simulink model "cdip_odq_sim"  (R2013a)
settings: Solver=ode4  SolverMode=SingleTasking  StartTime=0.0  StopTime=t_end  FixedStep=0.001  RelTol=1e-3
values from neighbouring files (symbols this model uses):
  dtheta_0 = 0    [p2c234_ex1_cdip_odq.m]    (also in p2c234_ex1_cdip_odq_custom.m; p2c244_ex3_cdip_sampled_data_lqr_sim.m; p2c244_ex3_cdip_sampled_data_lqr_sim_custom.m)
  dz_0 = 0    [p2c234_ex1_cdip_odq.m]    (also in p2c234_ex1_cdip_odq_custom.m; p2c244_ex3_cdip_sampled_data_lqr_sim.m; p2c244_ex3_cdip_sampled_data_lqr_sim_custom.m)
  K = - lqr(A,B,Q,R)    [p2c234_ex1_cdip_odq.m]    (also in p2c234_ex1_cdip_odq_custom.m; p2c244_ex3_cdip_sampled_data_lqr_sim.m; p2c244_ex3_cdip_sampled_data_lqr_sim_custom.m)
  theta_0 = pi/18    (= 0.174532925199)    [p2c234_ex1_cdip_odq.m]    (also in p2c234_ex1_cdip_odq_custom.m; p2c244_ex3_cdip_sampled_data_lqr_sim.m = 0.261799387799; p2c244_ex3_cdip_sampled_data_lqr_sim_custom.m = 0.261799387799)
  ts = 0.01    [p2c234_ex1_cdip_odq.m]    (also in p2c234_ex1_cdip_odq_custom.m; p2c242_ex2_cart_ipd.m = 0.025; p2c242_ex2_cart_ipd_custom.m = 0.025; p2c244_ex3_cdip_sampled_data_lqr_sim.m = 0.1)
  z_0 = 0    [p2c234_ex1_cdip_odq.m]    (also in p2c234_ex1_cdip_odq_custom.m; p2c244_ex3_cdip_sampled_data_lqr_sim.m; p2c244_ex3_cdip_sampled_data_lqr_sim_custom.m)
undefined symbols (not defined in the file or in its folder): ac, bc, g, Jp, lp, mp, mup, Sigma_Q
libraries: odqblock x1
settings Model: Creator=kawata  LastModifiedBy=kawata
settings SolverCC: AutoInsertRateTranBlk=on  InsertRTBMode=Always
settings DataIOCC: LimitDataPoints=off  SignalLoggingSaveFormat=ModelDataLogs
settings OptimizationCC: ExpressionDepthLimit=2147483647
settings DebuggingCC: FcnCallInpInsideContextMsg=UseLocalSettings
settings GRTTargetCC: CombineOutputUpdateFcns=off  GRTInterface=on

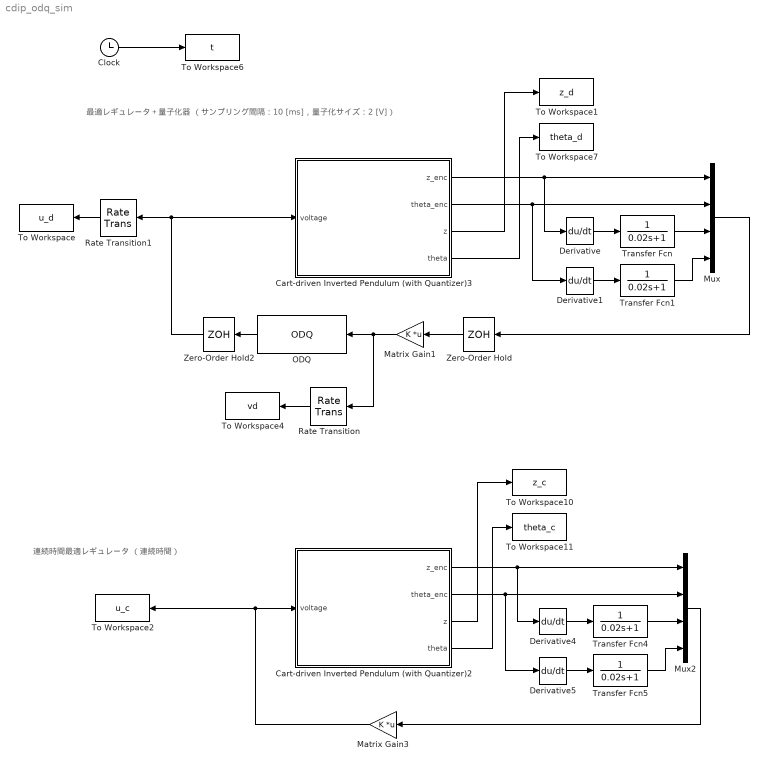
== system cdip_odq_sim ==
  note: 最適レギュレータ＋量子化器
      | （サンプリング間隔：10 [ms]，量子化サイズ：2 [V]）
  note: 連続時間最適レギュレータ
      | （連続時間）
  Cart-driven Inverted Pendulum (with Quantizer)2 : Subsystem
      mask Display: image(imread('cdip_photo.jpg'),'center')
  Cart-driven Inverted Pendulum (with Quantizer)3 : Subsystem
      mask Display: image(imread('cdip_photo.jpg'),'center')
  Clock : Clock
  Derivative{,1,4..5} (4 alike) : Derivative
  Matrix Gain1 : Gain  Gain=K  Multiplication=Matrix(K*u)  SaturateOnIntegerOverflow=on  OutDataTypeStr=Inherit: Same as input  ParamDataTypeStr=Inherit: Same as input
  Matrix Gain3 : Gain  Gain=K  Multiplication=Matrix(K*u)  SaturateOnIntegerOverflow=on  OutDataTypeStr=Inherit: Same as input  ParamDataTypeStr=Inherit: Same as input
  Mux : Mux
  Mux2 : Mux
  ODQ : odqblock/ODQ  A=Sigma_Q.a  B1=Sigma_Q.b1  B2=Sigma_Q.b2  C=Sigma_Q.c  d=d  Ts=ts
  Rate Transition : RateTransition  OutPortSampleTime=0.001
  Rate Transition1 : RateTransition  OutPortSampleTime=0.001
  To Workspace : ToWorkspace  VariableName=u_d  SampleTime=-1
  To Workspace1 : ToWorkspace  VariableName=z_d  SampleTime=-1
  To Workspace10 : ToWorkspace  VariableName=z_c  SampleTime=-1
  To Workspace11 : ToWorkspace  VariableName=theta_c  SampleTime=-1
  To Workspace2 : ToWorkspace  VariableName=u_c  SampleTime=0.001
  To Workspace4 : ToWorkspace  VariableName=vd  SampleTime=-1
  To Workspace6 : ToWorkspace  VariableName=t  SampleTime=-1
  To Workspace7 : ToWorkspace  VariableName=theta_d  SampleTime=-1
  Transfer Fcn{,1,4..5} (4 alike) : TransferFcn  Denominator=[0.02 1]
  Zero-Order Hold : ZeroOrderHold  SampleTime=ts
  Zero-Order Hold2 : ZeroOrderHold  SampleTime=ts
  wires:
  Zero-Order Hold/1 -> Matrix Gain1/1
  Zero-Order Hold2/1 -> Cart-driven Inverted Pendulum (with Quantizer)3/1(voltage), Rate Transition1/1
  Clock/1 -> To Workspace6/1
  ODQ/1 -> Zero-Order Hold2/1
  Matrix Gain1/1 -> ODQ/1, Rate Transition/1
  Rate Transition1/1 -> To Workspace/1
  Rate Transition/1 -> To Workspace4/1
  Mux/1 -> Zero-Order Hold/1
  Cart-driven Inverted Pendulum (with Quantizer)3/1(z_enc) -> Derivative/1, Mux/1
  Cart-driven Inverted Pendulum (with Quantizer)3/2(theta_enc) -> Derivative1/1, Mux/2
  Derivative/1 -> Transfer Fcn/1
  Transfer Fcn/1 -> Mux/3
  Transfer Fcn1/1 -> Mux/4
  Cart-driven Inverted Pendulum (with Quantizer)3/3(z) -> To Workspace1/1
  Cart-driven Inverted Pendulum (with Quantizer)3/4(theta) -> To Workspace7/1
  Derivative1/1 -> Transfer Fcn1/1
  Mux2/1 -> Matrix Gain3/1
  Matrix Gain3/1 -> To Workspace2/1, Cart-driven Inverted Pendulum (with Quantizer)2/1(voltage)
  Cart-driven Inverted Pendulum (with Quantizer)2/1(z_enc) -> Derivative4/1, Mux2/1
  Cart-driven Inverted Pendulum (with Quantizer)2/2(theta_enc) -> Derivative5/1, Mux2/2
  Derivative4/1 -> Transfer Fcn4/1
  Derivative5/1 -> Transfer Fcn5/1
  Transfer Fcn4/1 -> Mux2/3
  Transfer Fcn5/1 -> Mux2/4
  Cart-driven Inverted Pendulum (with Quantizer)2/3(z) -> To Workspace10/1
  Cart-driven Inverted Pendulum (with Quantizer)2/4(theta) -> To Workspace11/1

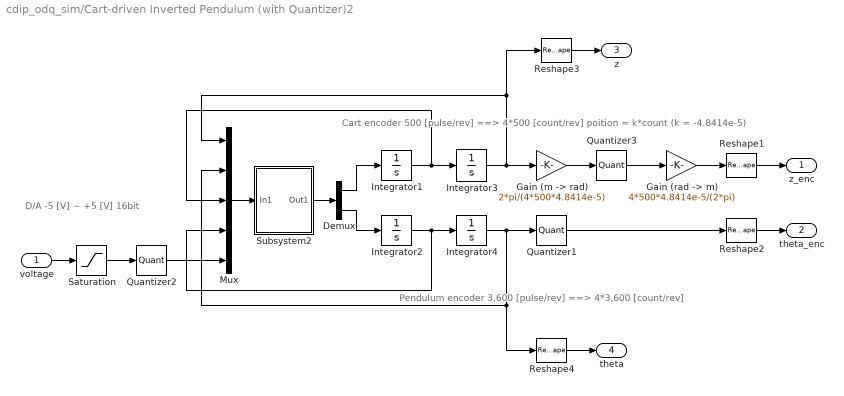
== system cdip_odq_sim/Cart-driven Inverted Pendulum (with Quantizer)2 ==
  note: Pendulum encoder
      |   3,600 [pulse/rev]  ==> 4*3,600 [count/rev]
  note: D/A
      |   -5 [V] ~ +5 [V]
      |  16bit
  note: Cart encoder
      |   500 [pulse/rev]  ==> 4*500 [count/rev]
      |   poition = k*count  (k = -4.8414e-5)
  voltage : Inport
  Demux : Demux  Outputs=2
  "Gain (m -> rad)" : Gain  Gain=2*pi/(4*500*4.8414e-5)  SaturateOnIntegerOverflow=on  OutDataTypeStr=Inherit: Same as input  ParamDataTypeStr=Inherit: Same as input
  "Gain (rad -> m)" : Gain  Gain=4*500*4.8414e-5/(2*pi)  SaturateOnIntegerOverflow=on  OutDataTypeStr=Inherit: Same as input  ParamDataTypeStr=Inherit: Same as input
  Integrator1 : Integrator  InitialCondition=dz_0
  Integrator2 : Integrator  InitialCondition=dtheta_0
  Integrator3 : Integrator  InitialCondition=z_0
  Integrator4 : Integrator  InitialCondition=theta_0
  Mux : Mux  Inputs=5
  Quantizer1 : Quantizer  QuantizationInterval=2*pi/(4*3600)
  Quantizer2 : Quantizer  QuantizationInterval=10/2^(16)
  Quantizer3 : Quantizer  QuantizationInterval=2*pi/(4*500)
  Reshape{1..4} (4 alike) : Reshape
  Saturation : Saturate  UpperLimit=5  LowerLimit=-5
  Subsystem2 : Subsystem
  z_enc : Outport
  theta_enc : Outport  Port=2
  z : Outport  Port=3
  theta : Outport  Port=4
  wires:
  Reshape2/1 -> theta_enc/1
  Reshape1/1 -> z_enc/1
  "Gain (rad -> m)"/1 -> Reshape1/1
  Quantizer3/1 -> "Gain (rad -> m)"/1
  "Gain (m -> rad)"/1 -> Quantizer3/1
  voltage/1 -> Saturation/1
  Integrator4/1 -> Quantizer1/1, Mux/2, Reshape4/1
  Integrator3/1 -> "Gain (m -> rad)"/1, Mux/1, Reshape3/1
  Integrator2/1 -> Integrator4/1, Mux/4
  Integrator1/1 -> Integrator3/1, Mux/3
  Demux/2 -> Integrator2/1
  Demux/1 -> Integrator1/1
  Mux/1 -> Subsystem2/1(In1)
  Subsystem2/1(Out1) -> Demux/1
  Quantizer1/1 -> Reshape2/1
  Quantizer2/1 -> Mux/5
  Saturation/1 -> Quantizer2/1
  Reshape3/1 -> z/1
  Reshape4/1 -> theta/1

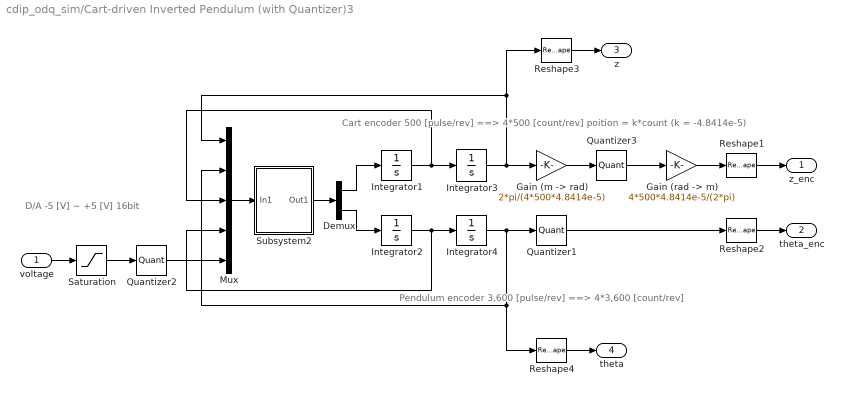
== system cdip_odq_sim/Cart-driven Inverted Pendulum (with Quantizer)3 ==
  note: Pendulum encoder
      |   3,600 [pulse/rev]  ==> 4*3,600 [count/rev]
  note: D/A
      |   -5 [V] ~ +5 [V]
      |  16bit
  note: Cart encoder
      |   500 [pulse/rev]  ==> 4*500 [count/rev]
      |   poition = k*count  (k = -4.8414e-5)
  voltage : Inport
  Demux : Demux  Outputs=2
  "Gain (m -> rad)" : Gain  Gain=2*pi/(4*500*4.8414e-5)  SaturateOnIntegerOverflow=on  OutDataTypeStr=Inherit: Same as input  ParamDataTypeStr=Inherit: Same as input
  "Gain (rad -> m)" : Gain  Gain=4*500*4.8414e-5/(2*pi)  SaturateOnIntegerOverflow=on  OutDataTypeStr=Inherit: Same as input  ParamDataTypeStr=Inherit: Same as input
  Integrator1 : Integrator  InitialCondition=dz_0
  Integrator2 : Integrator  InitialCondition=dtheta_0
  Integrator3 : Integrator  InitialCondition=z_0
  Integrator4 : Integrator  InitialCondition=theta_0
  Mux : Mux  Inputs=5
  Quantizer1 : Quantizer  QuantizationInterval=2*pi/(4*3600)
  Quantizer2 : Quantizer  QuantizationInterval=10/2^(16)
  Quantizer3 : Quantizer  QuantizationInterval=2*pi/(4*500)
  Reshape{1..4} (4 alike) : Reshape
  Saturation : Saturate  UpperLimit=5  LowerLimit=-5
  Subsystem2 : Subsystem
  z_enc : Outport
  theta_enc : Outport  Port=2
  z : Outport  Port=3
  theta : Outport  Port=4
  wires:
  Reshape2/1 -> theta_enc/1
  Reshape1/1 -> z_enc/1
  "Gain (rad -> m)"/1 -> Reshape1/1
  Quantizer3/1 -> "Gain (rad -> m)"/1
  "Gain (m -> rad)"/1 -> Quantizer3/1
  voltage/1 -> Saturation/1
  Integrator4/1 -> Quantizer1/1, Mux/2, Reshape4/1
  Integrator3/1 -> "Gain (m -> rad)"/1, Mux/1, Reshape3/1
  Integrator2/1 -> Integrator4/1, Mux/4
  Integrator1/1 -> Integrator3/1, Mux/3
  Demux/2 -> Integrator2/1
  Demux/1 -> Integrator1/1
  Mux/1 -> Subsystem2/1(In1)
  Subsystem2/1(Out1) -> Demux/1
  Quantizer1/1 -> Reshape2/1
  Quantizer2/1 -> Mux/5
  Saturation/1 -> Quantizer2/1
  Reshape3/1 -> z/1
  Reshape4/1 -> theta/1

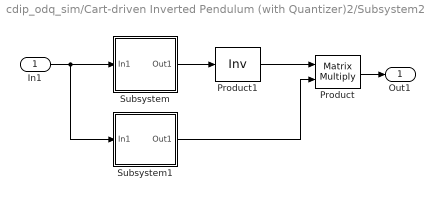
== system cdip_odq_sim/Cart-driven Inverted Pendulum (with Quantizer)2/Subsystem2 ==
  In1 : Inport
  Product : Product  Multiplication=Matrix(*)  SaturateOnIntegerOverflow=on  InputSameDT=on  OutDataTypeStr=Inherit: Same as first input
  Product1 : Product  Inputs=/  Multiplication=Matrix(*)  SaturateOnIntegerOverflow=on  InputSameDT=on  OutDataTypeStr=Inherit: Same as first input
  Subsystem : Subsystem
  Subsystem1 : Subsystem
  Out1 : Outport
  wires:
  Product/1 -> Out1/1
  In1/1 -> Subsystem1/1(In1), Subsystem/1(In1)
  Subsystem1/1(Out1) -> Product/2
  Product1/1 -> Product/1
  Subsystem/1(Out1) -> Product1/1

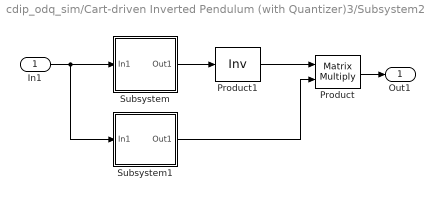
== system cdip_odq_sim/Cart-driven Inverted Pendulum (with Quantizer)3/Subsystem2 ==
  In1 : Inport
  Product : Product  Multiplication=Matrix(*)  SaturateOnIntegerOverflow=on  InputSameDT=on  OutDataTypeStr=Inherit: Same as first input
  Product1 : Product  Inputs=/  Multiplication=Matrix(*)  SaturateOnIntegerOverflow=on  InputSameDT=on  OutDataTypeStr=Inherit: Same as first input
  Subsystem : Subsystem
  Subsystem1 : Subsystem
  Out1 : Outport
  wires:
  Product/1 -> Out1/1
  In1/1 -> Subsystem1/1(In1), Subsystem/1(In1)
  Subsystem1/1(Out1) -> Product/2
  Product1/1 -> Product/1
  Subsystem/1(Out1) -> Product1/1

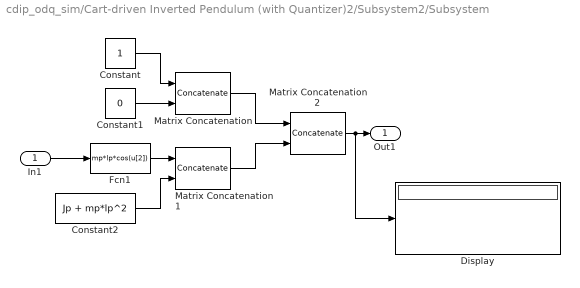
== system cdip_odq_sim/Cart-driven Inverted Pendulum (with Quantizer)2/Subsystem2/Subsystem ==
  In1 : Inport
  Constant : Constant
  Constant1 : Constant  Value=0
  Constant2 : Constant  Value=Jp + mp*lp^2
  Display : Display
  Fcn1 : Fcn  Expr=mp*lp*cos(u[2])
  Matrix Concatenation : Concatenate  Mode=Multidimensional array  ConcatenateDimension=2
  Matrix Concatenation1 : Concatenate  Mode=Multidimensional array  ConcatenateDimension=2
  Matrix Concatenation2 : Concatenate  Mode=Multidimensional array
  Out1 : Outport
  wires:
  Constant1/1 -> Matrix Concatenation/2
  Constant/1 -> Matrix Concatenation/1
  Matrix Concatenation2/1 -> Out1/1, Display/1
  Matrix Concatenation1/1 -> Matrix Concatenation2/2
  Matrix Concatenation/1 -> Matrix Concatenation2/1
  In1/1 -> Fcn1/1
  Fcn1/1 -> Matrix Concatenation1/1
  Constant2/1 -> Matrix Concatenation1/2

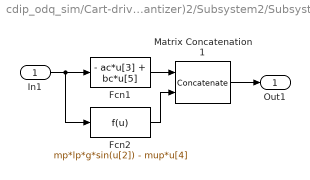
== system cdip_odq_sim/Cart-driven Inverted Pendulum (with Quantizer)2/Subsystem2/Subsystem1 ==
  In1 : Inport
  Fcn1 : Fcn  Expr=- ac*u[3] + bc*u[5]
  Fcn2 : Fcn  Expr=mp*lp*g*sin(u[2]) - mup*u[4]
  Matrix Concatenation1 : Concatenate  Mode=Multidimensional array
  Out1 : Outport
  wires:
  Matrix Concatenation1/1 -> Out1/1
  In1/1 -> Fcn1/1, Fcn2/1
  Fcn1/1 -> Matrix Concatenation1/1
  Fcn2/1 -> Matrix Concatenation1/2

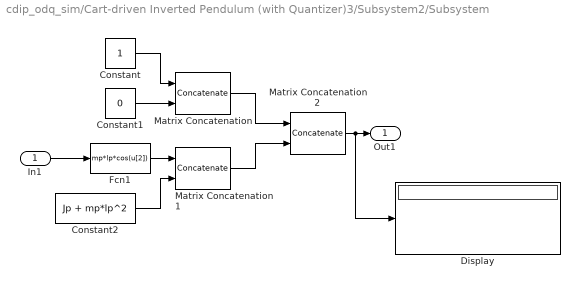
== system cdip_odq_sim/Cart-driven Inverted Pendulum (with Quantizer)3/Subsystem2/Subsystem ==
  In1 : Inport
  Constant : Constant
  Constant1 : Constant  Value=0
  Constant2 : Constant  Value=Jp + mp*lp^2
  Display : Display
  Fcn1 : Fcn  Expr=mp*lp*cos(u[2])
  Matrix Concatenation : Concatenate  Mode=Multidimensional array  ConcatenateDimension=2
  Matrix Concatenation1 : Concatenate  Mode=Multidimensional array  ConcatenateDimension=2
  Matrix Concatenation2 : Concatenate  Mode=Multidimensional array
  Out1 : Outport
  wires:
  Constant1/1 -> Matrix Concatenation/2
  Constant/1 -> Matrix Concatenation/1
  Matrix Concatenation2/1 -> Out1/1, Display/1
  Matrix Concatenation1/1 -> Matrix Concatenation2/2
  Matrix Concatenation/1 -> Matrix Concatenation2/1
  In1/1 -> Fcn1/1
  Fcn1/1 -> Matrix Concatenation1/1
  Constant2/1 -> Matrix Concatenation1/2

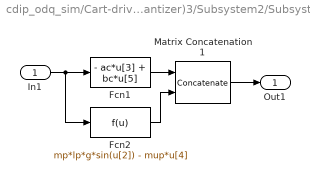
== system cdip_odq_sim/Cart-driven Inverted Pendulum (with Quantizer)3/Subsystem2/Subsystem1 ==
  In1 : Inport
  Fcn1 : Fcn  Expr=- ac*u[3] + bc*u[5]
  Fcn2 : Fcn  Expr=mp*lp*g*sin(u[2]) - mup*u[4]
  Matrix Concatenation1 : Concatenate  Mode=Multidimensional array
  Out1 : Outport
  wires:
  Matrix Concatenation1/1 -> Out1/1
  In1/1 -> Fcn1/1, Fcn2/1
  Fcn1/1 -> Matrix Concatenation1/1
  Fcn2/1 -> Matrix Concatenation1/2
